simulink model "Bai5A_3"  (R2015a)
settings: Solver=ode45  StartTime=0.0  StopTime=10.0  RelTol=1e-3
libraries: commchan3 x1, commsink2 x1, commutil2 x1, commfilt2 x1, dspstat3 x1, commrandsrc2 x1
settings Model: Creator=Trong  LastModifiedBy=Trong

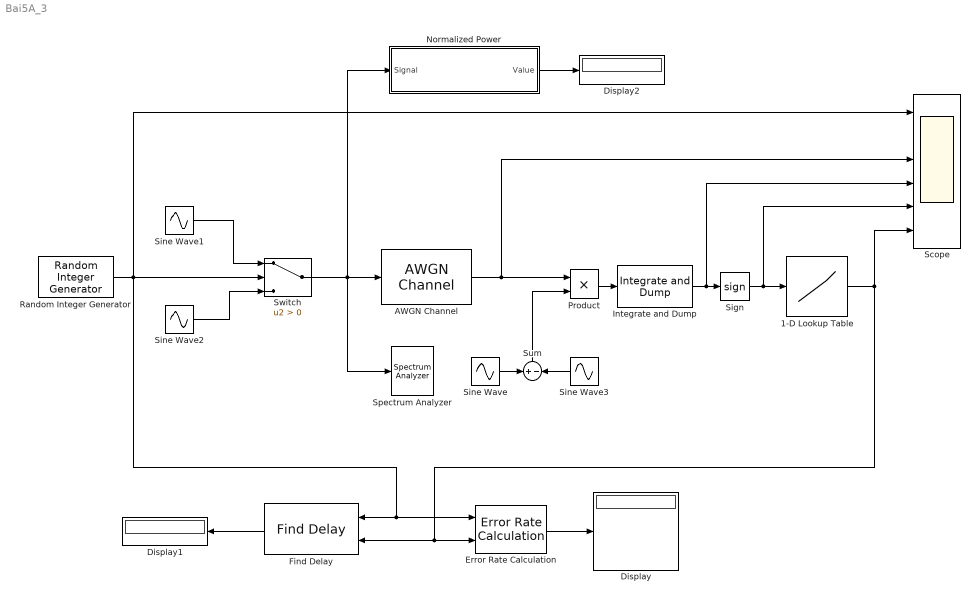
== system Bai5A_3 ==
  1-D Lookup Table : Lookup_n-D  NumberOfTableDimensions=1  BreakpointsForDimension1=[-5:5]  Table=tanh([-5:5])  InternalRulePriority=Speed  RndMeth=Simplest  InputSameDT=on
  AWGN Channel : commchan3/AWGN Channel  InputProcessing=Columns as channels (frame based)  seed=67  noiseMode="Signal to noise ratio  (Eb/No)"  EbNodB=10  EsNodB=10  SNRdB=10  bitsPerSym=1  Ps=1  Tsym=1  variance=1
  Display : Display
  Display1 : Display
  Display2 : Display
  Error Rate Calculation : commsink2/Error Rate Calculation  N=0  st_delay=0  cp_mode=Entire frame  subframe=[]  PMode=Port  WsName=ErrorVec  RsMode2=off  stop=off  numErr=100  maxBits=1e6
  Find Delay : commutil2/Find Delay  corrLength=200  chgSigOP=off  stopUpdate=off  numConstDelay=3
  Integrate and Dump : commfilt2/Integrate and Dump  obssamples=8  offsetsamples=0  nodump=off  roundingMode=Floor  overflowMode=off
  Normalized Power : Subsystem
  Product : Product
  Random Integer Generator : commrandsrc2/Random Integer Generator  mul=8  seed=37  Ts=1  frameBased=off  sampPerFrame=1  orient=off  outDataType=double
  Scope : Scope  NumInputPorts=6
      settings: YMin=-5~-5~-5~-5~-5~-5  YMax=5~5~5~5~5~5
  Sign : Signum
  Sine Wave{,1..3} (4 alike) : Sin  SampleTime=0
  Spectrum Analyzer : SpectrumAnalyzer
  Sum : Sum  Inputs=+-
  Switch : Switch  Criteria=u2 > Threshold
  wires:
  AWGN Channel/1 -> Scope/3, Product/1
  Product/1 -> Integrate and Dump/1
  Integrate and Dump/1 -> Scope/4, Sign/1
  Sign/1 -> Scope/5, 1-D Lookup Table/1
  Error Rate Calculation/1 -> Display/1
  Random Integer Generator/1 -> Find Delay/1, Error Rate Calculation/1, Switch/2, Scope/1
  1-D Lookup Table/1 -> Error Rate Calculation/2, Find Delay/2, Scope/6
  Find Delay/1 -> Display1/1
  Normalized Power/1(Value) -> Display2/1
  Switch/1 -> Spectrum Analyzer/1, Normalized Power/1(Signal), AWGN Channel/1
  Sine Wave1/1 -> Switch/1
  Sine Wave2/1 -> Switch/3
  Sine Wave/1 -> Sum/1
  Sine Wave3/1 -> Sum/2
  Sum/1 -> Product/2

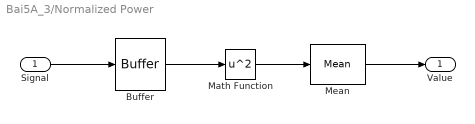
== system Bai5A_3/Normalized Power ==
  Signal : Inport
  Buffer : Buffer  TreatMby1Signals=One channel
  Math Function : Math  Operator=square  SaturateOnIntegerOverflow=on
  Mean : dspstat3/Mean  run=off  reset_popup=None  InputProcessing=Columns as channels (frame based)  directionMode=Each column  dimension=1  treatSBRowAsCol=off  roiEnable=off  roiType=Rectangles  roiPortion=Entire ROI  roiOutput=Individual statistics for each ROI  roiFlag=off  outputDataTypeStr=Inherit: Same as accumulator  outputLastDataTypeStr=Inherit: Same as accumulator  outputMin=[]  outputMax=[]  roundingMode=Floor  overflowMode=off
  Value : Outport
  wires:
  Signal/1 -> Buffer/1
  Buffer/1 -> Math Function/1
  Mean/1 -> Value/1
  Math Function/1 -> Mean/1
